simulink model "rpihil"  (R2025b)
settings: Solver=FixedStepDiscrete  StartTime=0.0  StopTime=inf  FixedStep=0.002  RelTol=1e-3  EnableMultiTasking=on
libraries: quarc_library x12
settings Model: SimulationMode=external  ExtModeTrigDuration=10000  Creator=epicm  LastModifiedBy=Cera Wang
settings SolverCC: AlgebraicLoopSolver=TrustRegion  PositivePriorityOrder=on
settings DataIOCC: ReturnWorkspaceOutputs=off
settings DebuggingCC: UnconnectedInputMsg=warning  UnconnectedOutputMsg=warning  UnconnectedLineMsg=warning  ArithmeticOperatorsInVariantConditions=warning
settings HardwareCC: ProdBitPerLong=64.0  ProdLargestAtomicInteger=LongLong  ProdLargestAtomicFloat=Double  ProdLongLongMode=on  ProdHWDeviceType=ARM Compatible->ARM 64-bit (LP64)
settings ModelReferenceCC: EnableRefExpFcnMdlSchedulingChecks=on
settings SFSimCC: SimUseLocalCustomCode=off  CustomCodeUndefinedFunction=UseInterfaceOnly
settings RTWCC: SystemTargetFile=quarc_linux_pi_arm64.tlc  TemplateMakefile=quarc_default_tmf  RTWUseLocalCustomCode=off  Toolchain=QUARC linux_pi_arm64 | gmake (64-bit Windows)  BuildConfiguration=Faster Runs  GPUComputeCapability=3.5  Description=QUARC Linux Raspberry Pi Arm64 Target (QBot Platform Alpha) Using Toolchain
settings CodeAppCC: StateflowObjectComments=on
settings STFCustomTargetCC: SystemTargetFile=quarc_linux_pi_arm64.tlc  UseToolchainInfoCompliant=on  StripSymbols=off  MinimumThreadPriority=20.0
settings GRTTargetCC: ExtMode=on  ExtModeMexFile=quarc_comm  ExtModeMexArgs='-w -d /tmp -uri %u'  TargetLangStandard=C89/C90 (ANSI)  ParMdlRefBuildCompliant=off  CompOptLevelCompliant=off  CombineOutputUpdateFcns=off  MatFileLogging=off  CPPClassGenCompliant=off  GRTInterface=on
settings ConfigComp: CovMetricSettings=dswe

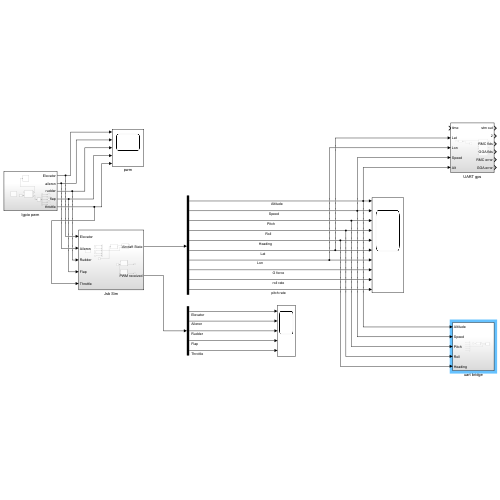
[thumbnail: Simulink's stored preview of the top-level diagram]
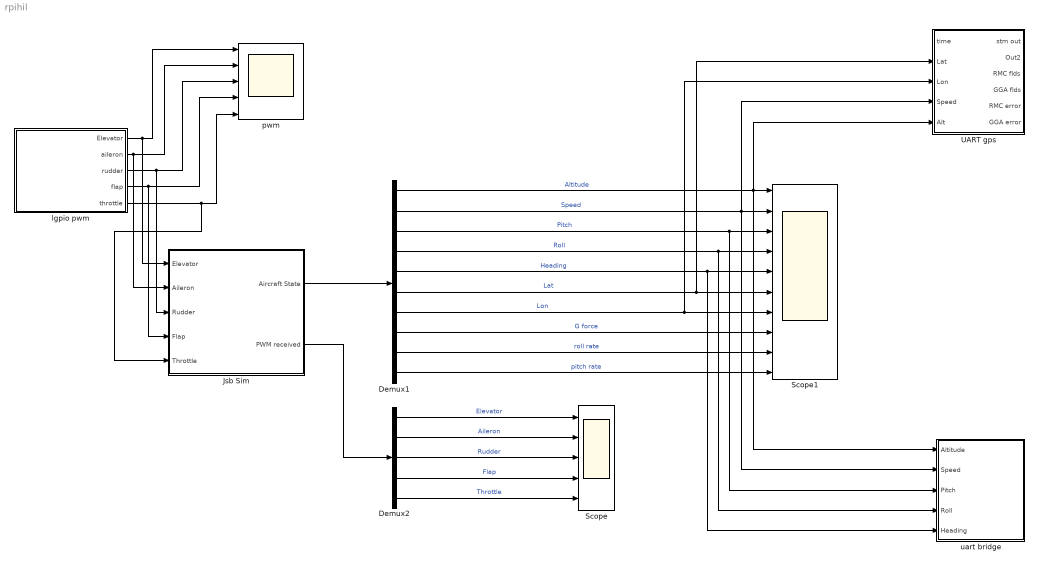
== system rpihil ==
  Demux1 : Demux  Outputs=10
  Demux2 : Demux  Outputs=5
  Jsb Sim : Subsystem
  Scope : Scope  NumInputPorts=5
      settings: ActiveDisplayYMinimum=-11.225752447687823  ActiveDisplayYMaximum=12.45905740212261  DataLoggingVariableName=ScopeData2
  Scope1 : Scope  NumInputPorts=10
      settings: ActiveDisplayYMinimum=-1.3561505356268164E+292  ActiveDisplayYMaximum=1.220535482064135E+293
  UART gps : Subsystem
  lgpio pwm : Subsystem
  pwm : Scope  NumInputPorts=5
      settings: ActiveDisplayYMinimum=-6.2067872171984462  ActiveDisplayYMaximum=10.079398269933932
  uart bridge : Subsystem
  wires:
  lgpio pwm/1(Elevator) -> Jsb Sim/1(Elevator), pwm/1
  lgpio pwm/2(aileron) -> Jsb Sim/2(Aileron), pwm/2
  lgpio pwm/4(flap) -> pwm/4, Jsb Sim/4(Flap)
  lgpio pwm/3(rudder) -> Jsb Sim/3(Rudder), pwm/3
  Demux1/1 -> uart bridge/1(Altitude), UART gps/5(Alt), Scope1/1  "Altitude"
  Demux1/2 -> uart bridge/2(Speed), UART gps/4(Speed), Scope1/2  "Speed"
  Demux1/3 -> uart bridge/3(Pitch), Scope1/3  "Pitch"
  Demux1/4 -> uart bridge/4(Roll), Scope1/4  "Roll"
  Demux1/5 -> uart bridge/5(Heading), Scope1/5  "Heading"
  Demux1/6 -> UART gps/2(Lat), Scope1/6  "Lat"
  Demux1/8 -> Scope1/8  "G force"
  Demux1/9 -> Scope1/9  "roll rate"
  Demux1/10 -> Scope1/10  "pitch rate"
  Demux1/7 -> UART gps/3(Lon), Scope1/7  "Lon"
  Jsb Sim/1(Aircraft State) -> Demux1/1
  lgpio pwm/5(throttle) -> Jsb Sim/5(Throttle), pwm/5
  Jsb Sim/2(PWM received) -> Demux2/1
  Demux2/1 -> Scope/1  "Elevator"
  Demux2/2 -> Scope/2  "Aileron"
  Demux2/3 -> Scope/3  "Rudder"
  Demux2/4 -> Scope/4  "Flap"
  Demux2/5 -> Scope/5  "Throttle"

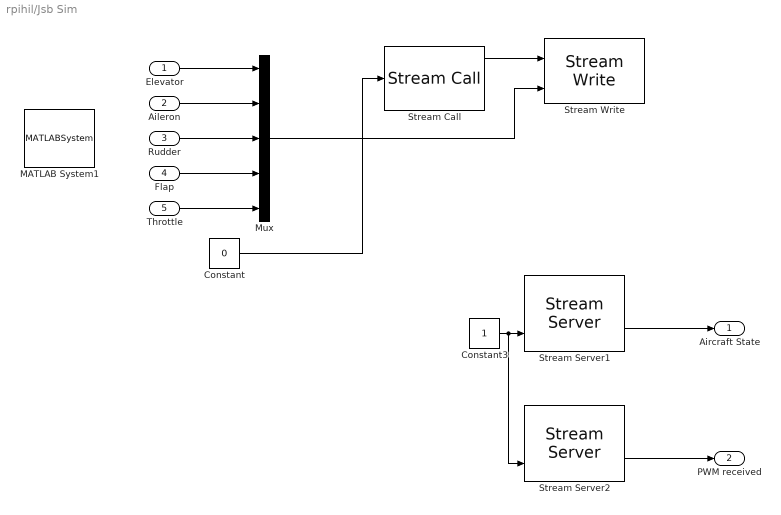
== system rpihil/Jsb Sim ==
  Elevator : Inport
  Aileron : Inport  Port=2
  Rudder : Inport  Port=3
  Flap : Inport  Port=4
  Throttle : Inport  Port=5
  Constant : Constant  Value=0
  Constant3 : Constant
  MATLAB System1 : MATLABSystem  System=flightserver  SimulateUsing=Code generation
      mask Type: flightserver
  Mux : Mux  Inputs=5
  Stream Call : quarc_library/Communications/Intermediate/Stream Call  uri_source=Specify via dialog (do not evaluate)  uri=udp://127.0.0.1:18000  send_buffer_size=8000  receive_buffer_size=8000  byte_order=little endian (Intel - LSB first)  sample_time=qc_get_step_size  non_blocking=on  active=off
      settings: AttributesFormatString="\"udp://127.0.0.1:18000\""  SourceProductName=QUARC Targets
  Stream Server1 : quarc_library/Communications/Basic/Stream Server  uri_source=Specify via dialog (do not evaluate)  uri=udp://127.0.0.1:18001  send_buffer_size=8000  receive_buffer_size=8000  byte_order=little endian (Intel - LSB first)  optimization=Minimum latency  send_options=Send all data  receive_options=Receive all data  default_value=[0, 0, 0, 0, 0, 0, 0, 0, 0, 0]  sample_time=qc_get_step_size  active=off  implementation=Use blocking I/O in a separate thread  send_fifo_size=1000  receive_fifo_size=1000  send_priority=0  receive_priority=0  send_dimensions=off  receive_dimensions=off  max_dimensions=4  data_type=Inherited via back propagation  type_expr=BusObject
      settings: AttributesFormatString="\"udp://127.0.0.1:18001\""
  Stream Server2 : quarc_library/Communications/Basic/Stream Server  uri_source=Specify via dialog (do not evaluate)  uri=udp://127.0.0.1:18005  send_buffer_size=8000  receive_buffer_size=8000  byte_order=little endian (Intel - LSB first)  optimization=Minimum latency  send_options=Send all data  receive_options=Receive all data  default_value=[0, 0, 0, 0, 0, 0, 0, 0, 0, 0]  sample_time=qc_get_step_size  active=off  implementation=Use blocking I/O in a separate thread  send_fifo_size=1000  receive_fifo_size=1000  send_priority=0  receive_priority=0  send_dimensions=off  receive_dimensions=off  max_dimensions=4  data_type=Inherited via back propagation  type_expr=BusObject
      settings: AttributesFormatString="\"udp://127.0.0.1:18005\""
  Stream Write : quarc_library/Communications/Intermediate/Stream Write  optimization=Minimizing latency  send_dims=off
      settings: SourceProductName=QUARC Targets
  Aircraft State : Outport  PortDimensions=10
  PWM received : Outport  Port=2  PortDimensions=10
  wires:
  Aileron/1 -> Mux/2
  Elevator/1 -> Mux/1
  Rudder/1 -> Mux/3
  Throttle/1 -> Mux/5
  Flap/1 -> Mux/4
  Stream Call/1 -> Stream Write/1
  Mux/1 -> Stream Write/2
  Constant/1 -> Stream Call/1
  Stream Server1/4 -> Aircraft State/1
  Constant3/1 -> Stream Server2/2, Stream Server1/2
  Stream Server2/4 -> PWM received/1

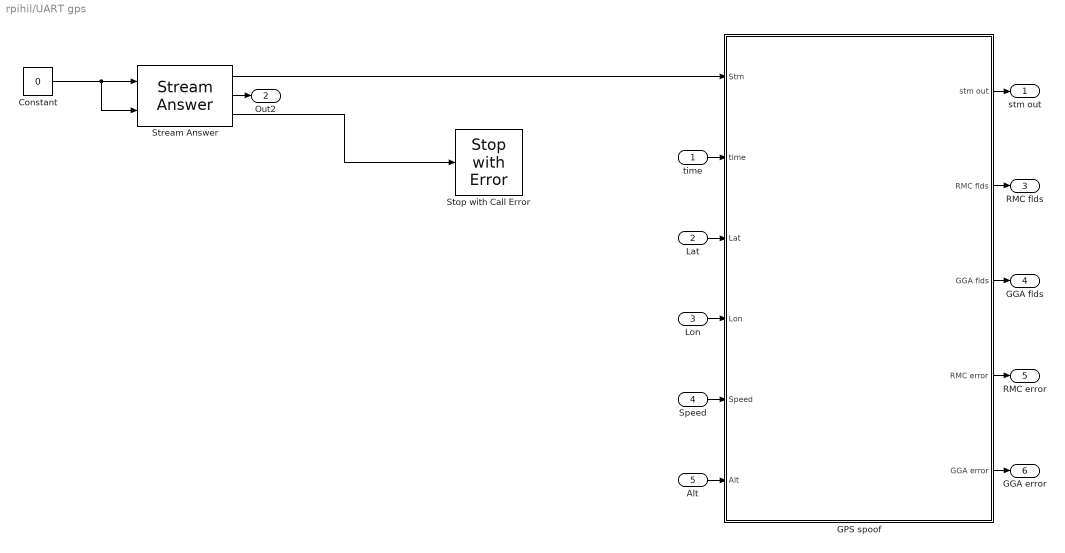
== system rpihil/UART gps ==
  time : Inport
  Lat : Inport  Port=2
  Lon : Inport  Port=3
  Speed : Inport  Port=4
  Alt : Inport  Port=5
  Constant : Constant  Value=0
  GPS spoof : Subsystem
  Stop with Call Error : quarc_library/Sinks/Error Handling/Stop with Error  message_type=Interpret input as error code  message=Error occurred
      settings: SourceProductName=QUARC Targets
  Stream Answer : quarc_library/Communications/Intermediate/Stream Answer  uri_source=Specify via dialog (do not evaluate)  uri=serial://localhost:0?baud=9600,word=8,parity=none,stop=1,flow=none  send_buffer_size=8000  receive_buffer_size=8000  byte_order=little endian (Intel - LSB first)  sample_time=qc_get_step_size  active=off
      settings: AttributesFormatString="\"serial://localhost:0?baud=9600,word=8,parity=none,stop=1,flow=none\""  SourceProductName=QUARC Targets
  stm out : Outport
  Out2 : Outport  Port=2
  RMC flds : Outport  Port=3
  GGA flds : Outport  Port=4
  RMC error : Outport  Port=5
  GGA error : Outport  Port=6
  wires:
  Constant/1 -> Stream Answer/1, Stream Answer/2
  GPS spoof/5(GGA error) -> GGA error/1
  Stream Answer/2 -> Out2/1
  GPS spoof/1(stm out) -> stm out/1
  GPS spoof/2(RMC flds) -> RMC flds/1
  Stream Answer/3 -> Stop with Call Error/1
  Stream Answer/1 -> GPS spoof/1(Stm)
  Lon/1 -> GPS spoof/4(Lon)
  time/1 -> GPS spoof/2(time)
  GPS spoof/3(GGA flds) -> GGA flds/1
  GPS spoof/4(RMC error) -> RMC error/1
  Speed/1 -> GPS spoof/5(Speed)
  Alt/1 -> GPS spoof/6(Alt)
  Lat/1 -> GPS spoof/3(Lat)

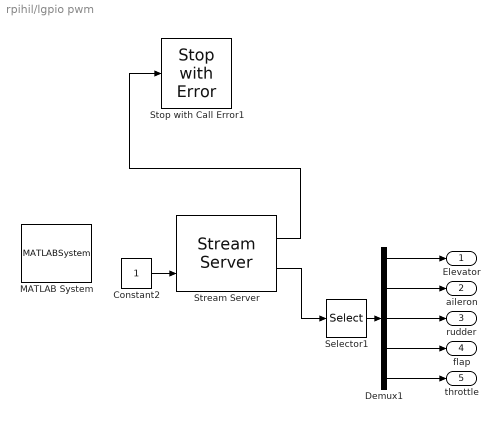
== system rpihil/lgpio pwm ==
  Constant2 : Constant
  Demux1 : Demux  Outputs=5
  MATLAB System : MATLABSystem  System=PigpioLauncher  SimulateUsing=Code generation
      mask Type: PigpioLauncher
  Selector1 : Selector  InputPortWidth=5  IndexOptions=Index vector (dialog)  Indices=[1 2 3 4 5]  OutputSizes=1
  Stop with Call Error1 : quarc_library/Sinks/Error Handling/Stop with Error  message_type=Interpret input as error code  message=Error occurred
      settings: SourceProductName=QUARC Targets
  Stream Server : quarc_library/Communications/Basic/Stream Server  uri_source=Specify via dialog (do not evaluate)  uri=udp://:50005  send_buffer_size=8000  receive_buffer_size=8000  byte_order=little endian (Intel - LSB first)  optimization=Minimum latency  send_options=Send all data  receive_options=Receive all data  default_value=[0 0 0 0 0]  sample_time=qc_get_step_size  active=off  implementation=Use blocking I/O in a separate thread  send_fifo_size=1000  receive_fifo_size=1000  send_priority=0  receive_priority=0  send_dimensions=off  receive_dimensions=off  max_dimensions=5  data_type=Inherited via back propagation  type_expr=BusObject
      settings: AttributesFormatString="\"udp://:50005\""
  Elevator : Outport
  aileron : Outport  Port=2
  rudder : Outport  Port=3
  flap : Outport  Port=4
  throttle : Outport  Port=5
  wires:
  Stream Server/4 -> Selector1/1
  Selector1/1 -> Demux1/1
  Constant2/1 -> Stream Server/2
  Demux1/5 -> throttle/1
  Demux1/4 -> flap/1
  Demux1/3 -> rudder/1
  Demux1/2 -> aileron/1
  Demux1/1 -> Elevator/1
  Stream Server/2 -> Stop with Call Error1/1

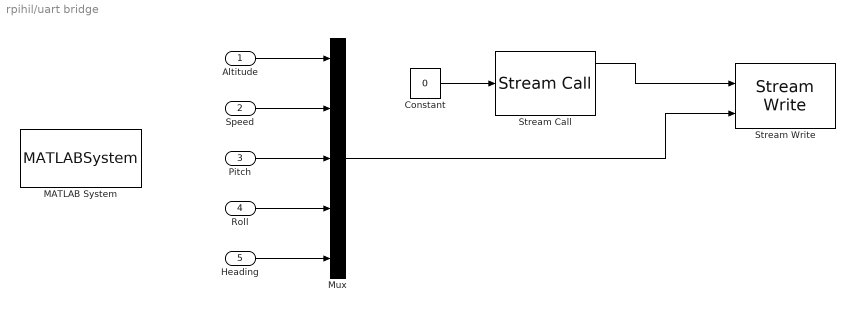
== system rpihil/uart bridge ==
  Altitude : Inport
  Speed : Inport  Port=2
  Pitch : Inport  Port=3
  Roll : Inport  Port=4
  Heading : Inport  Port=5
  Constant : Constant  Value=0
  MATLAB System : MATLABSystem  System=UartBridgeLauncher  SimulateUsing=Code generation
      mask Type: UartBridgeLauncher
  Mux : Mux  Inputs=5
  Stream Call : quarc_library/Communications/Intermediate/Stream Call  uri_source=Specify via dialog (do not evaluate)  uri=udp://127.0.0.1:18002  send_buffer_size=8000  receive_buffer_size=8000  byte_order=little endian (Intel - LSB first)  sample_time=qc_get_step_size  non_blocking=on  active=off
      settings: AttributesFormatString="\"udp://127.0.0.1:18002\""  SourceProductName=QUARC Targets
  Stream Write : quarc_library/Communications/Intermediate/Stream Write  optimization=Minimizing latency  send_dims=off
      settings: SourceProductName=QUARC Targets
  wires:
  Altitude/1 -> Mux/1
  Speed/1 -> Mux/2
  Pitch/1 -> Mux/3
  Roll/1 -> Mux/4
  Heading/1 -> Mux/5
  Constant/1 -> Stream Call/1
  Stream Call/1 -> Stream Write/1
  Mux/1 -> Stream Write/2

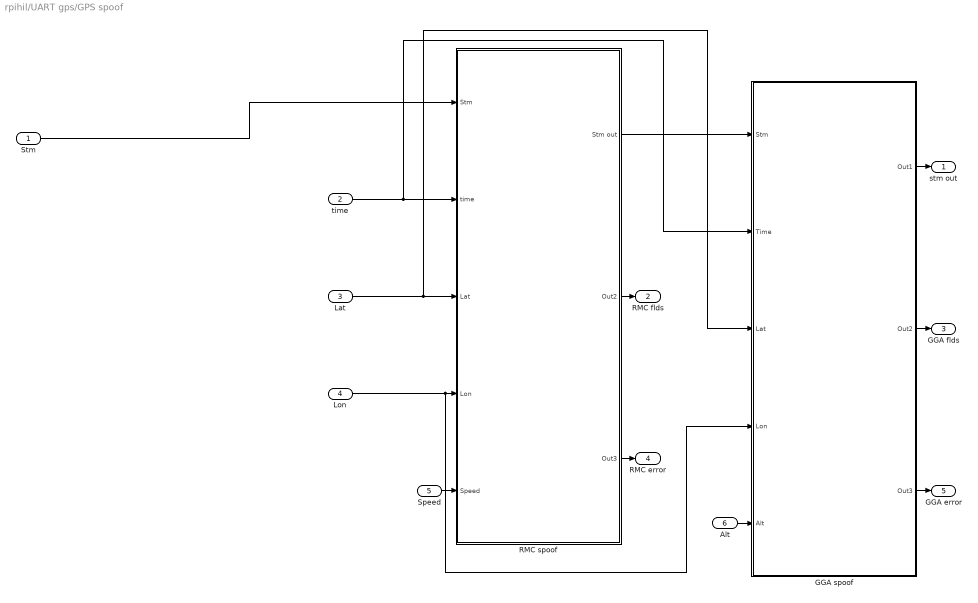
== system rpihil/UART gps/GPS spoof ==
  Stm : Inport
  time : Inport  Port=2
  Lat : Inport  Port=3
  Lon : Inport  Port=4
  Speed : Inport  Port=5
  Alt : Inport  Port=6
  GGA spoof : Subsystem
  RMC spoof : Subsystem
  stm out : Outport
  RMC flds : Outport  Port=2
  GGA flds : Outport  Port=3
  RMC error : Outport  Port=4
  GGA error : Outport  Port=5
  wires:
  RMC spoof/1(Stm out) -> GGA spoof/1(Stm)
  RMC spoof/3(Out3) -> RMC error/1
  Stm/1 -> RMC spoof/1(Stm)
  Speed/1 -> RMC spoof/5(Speed)
  time/1 -> GGA spoof/2(Time), RMC spoof/2(time)
  Lat/1 -> GGA spoof/3(Lat), RMC spoof/3(Lat)
  RMC spoof/2(Out2) -> RMC flds/1
  Alt/1 -> GGA spoof/5(Alt)
  GGA spoof/1(Out1) -> stm out/1
  GGA spoof/3(Out3) -> GGA error/1
  GGA spoof/2(Out2) -> GGA flds/1
  Lon/1 -> GGA spoof/4(Lon), RMC spoof/4(Lon)

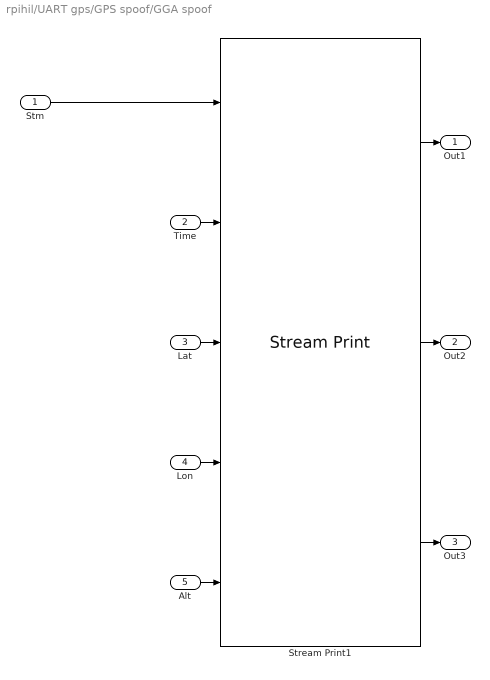
== system rpihil/UART gps/GPS spoof/GGA spoof ==
  Stm : Inport
  Time : Inport  Port=2
  Lat : Inport  Port=3
  Lon : Inport  Port=4
  Alt : Inport  Port=5
  Stream Print1 : quarc_library/Communications/Advanced/Stream Print  format_string=$GPGGA,%09.2f,%010.5f,N,%011.5f,E,1,12,1.01,%.1f,M,48,M,  max_code_units=80
      settings: SourceProductName=QUARC Targets
  Out1 : Outport
  Out2 : Outport  Port=2
  Out3 : Outport  Port=3
  wires:
  Stm/1 -> Stream Print1/1
  Alt/1 -> Stream Print1/5
  Lat/1 -> Stream Print1/3
  Time/1 -> Stream Print1/2
  Lon/1 -> Stream Print1/4
  Stream Print1/1 -> Out1/1
  Stream Print1/3 -> Out3/1
  Stream Print1/2 -> Out2/1

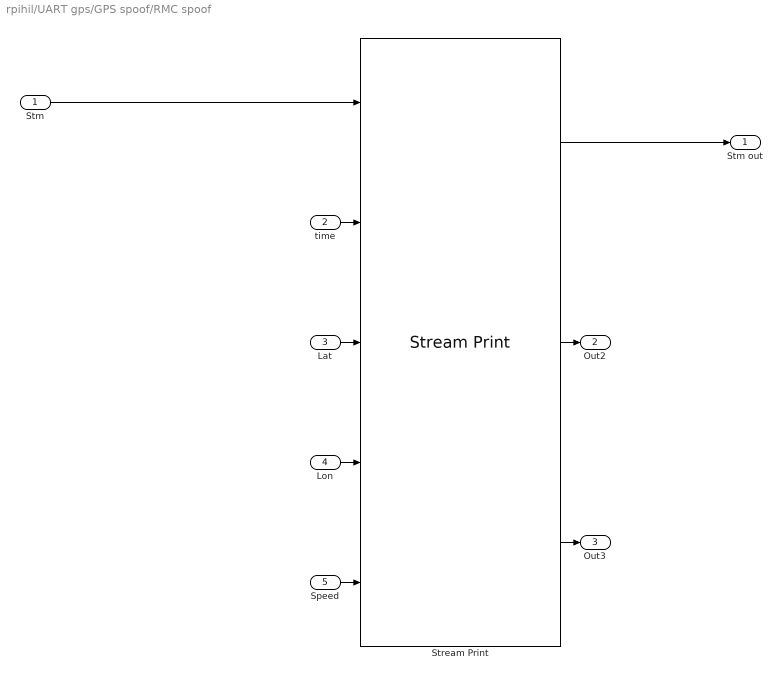
== system rpihil/UART gps/GPS spoof/RMC spoof ==
  Stm : Inport
  time : Inport  Port=2
  Lat : Inport  Port=3
  Lon : Inport  Port=4
  Speed : Inport  Port=5
  Stream Print : quarc_library/Communications/Advanced/Stream Print  format_string=$GPRMC,%09.2f,A,%010.5f,N,%011.5f,E,%.3f,  max_code_units=80
      settings: SourceProductName=QUARC Targets
  Stm out : Outport
  Out2 : Outport  Port=2
  Out3 : Outport  Port=3
  wires:
  Stm/1 -> Stream Print/1
  Lat/1 -> Stream Print/3
  Stream Print/1 -> Stm out/1
  Lon/1 -> Stream Print/4
  Speed/1 -> Stream Print/5
  Stream Print/3 -> Out3/1
  time/1 -> Stream Print/2
  Stream Print/2 -> Out2/1
